simulink model "SalirClaseConObstaculos"  (R2023b)
settings: Solver=FixedStepDiscrete  StartTime=0.0  StopTime=100  FixedStep=0.01  RelTol=1e-3  EnableMultiTasking=on
model workspace (MAT data in the model file):
  baldosa = 0.48
  d = 0.2625
libraries: robotalgslib x1
settings Model: ExtModeTrigDuration=2  Creator=Usuario_UMA  LastModifiedBy=pablo
settings SolverCC: AlgebraicLoopSolver=TrustRegion
settings OptimizationCC: EnhancedBackFolding=on  PassReuseOutputArgsAs=Individual arguments  ZeroExternalMemoryAtStartup=off  ZeroInternalMemoryAtStartup=off  MaxStackSize=64  OptimizeBlockOrder=speed  DifferentSizesBufferReuse=on  EfficientTunableParamExpr=on
settings DebuggingCC: ParameterTunabilityLossMsg=error  UnconnectedInputMsg=warning  UnconnectedOutputMsg=warning  UnconnectedLineMsg=warning
settings HardwareCC: ProdBitPerInt=16  ProdBitPerPointer=16  ProdBitPerSizeT=16  ProdBitPerPtrDiffT=16  ProdLargestAtomicFloat=None  ProdWordSize=8  ProdHWDeviceType=Atmel->AVR  UseEmbeddedCoderFeatures=off  UseSimulinkCoderFeatures=off
settings ModelReferenceCC: EnableRefExpFcnMdlSchedulingChecks=on
settings SFSimCC: MATLABDynamicMemAlloc=off
settings RTWCC: Description=Embedded Coder  SystemTargetFile=ert.tlc  HardwareBoard=Arduino Mega 2560  TemplateMakefile=ert_default_tmf  Toolchain=Arduino AVR  BuildConfiguration=Faster Runs  DLArmComputeVersion=19.05
settings CodeAppCC: ForceParamTrailComments=on  IgnoreCustomStorageClasses=off  OperatorAnnotations=on  SimulinkDataObjDesc=on  SFDataObjDesc=on  InsertBlockDesc=on
settings ERTTargetCC: SupportContinuousTime=on  SupportNonInlinedSFcns=on  SupportVariableSizeSignals=on  ExtModeTransport=3  ExtModeStaticAlloc=on  ExtModeAutomaticAllocSize=off  ExtModeStaticAllocSize=2048  ExtModeMexFile=ext_xcp  ExtModeIntrfLevel=Level2 - Open

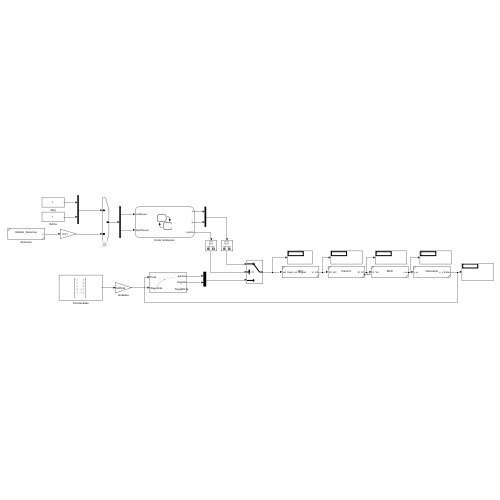
[thumbnail: Simulink's stored preview of the top-level diagram]
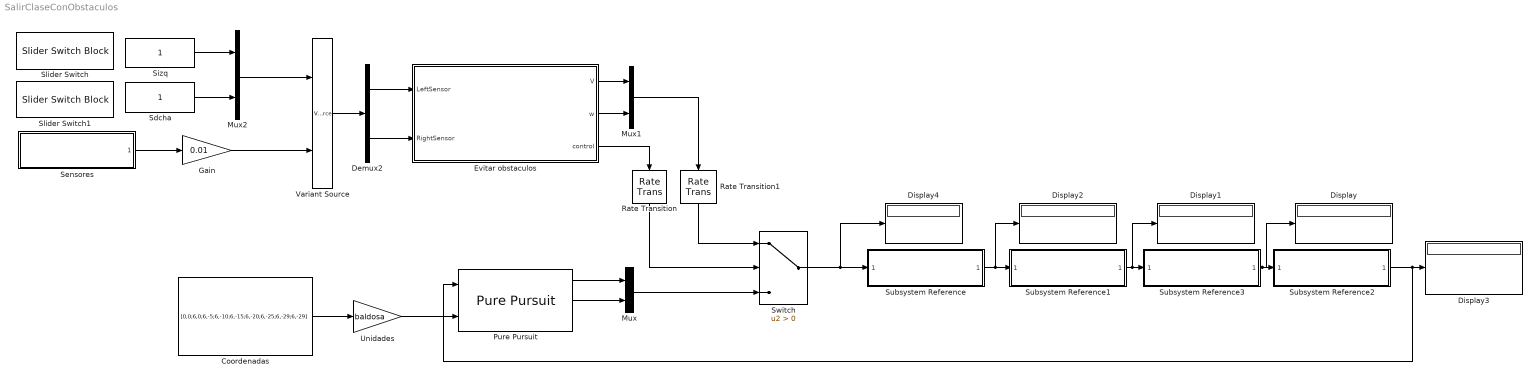
== system SalirClaseConObstaculos ==
  Coordenadas : Constant  Value=[0,0;6,0;6,-5;6,-10;6,-15;6,-20;6,-25;6,-29;6,-29]
  Demux2 : Demux  Outputs=2
  Display{,1..4} (5 alike) : Display
  Evitar obstaculos : Stateflow chart  TreatAsAtomicUnit=on
  Gain : Gain  Gain=0.01  OutDataTypeStr=double
  Mux : Mux  Inputs=2
  Mux1 : Mux  Inputs=2
  Mux2 : Mux  Inputs=2
  Pure Pursuit : robotalgslib/Pure Pursuit  DesiredLinearVelocity=0.205  MaxAngularVelocity=1.5  LookaheadDistance=0.2  TargetDirPort=on  SimulateUsing=Code generation
      settings: LibrarySourceBlock=navlib/Control Algorithms/Pure Pursuit
  Rate Transition : RateTransition
  Rate Transition1 : RateTransition
  Sdcha : Constant
  Sensores : Subsystem  ReferencedSubsystem=Modelo_Sensores
  Sizq : Constant
  Slider Switch : SliderSwitchBlock
      settings: Values={{'Libre', 'Obstaculo'}, [1 0.29]}
  Slider Switch1 : SliderSwitchBlock
      settings: Values={{'Libre', 'Obstaculo'}, [1 0.29]}
  Subsystem Reference : Subsystem  ReferencedSubsystem=MCI
  Subsystem Reference1 : Subsystem  ReferencedSubsystem=PieroCV
  Subsystem Reference2 : Subsystem  ReferencedSubsystem=Odometria
  Subsystem Reference3 : Subsystem  ReferencedSubsystem=MCD
  Switch : Switch  Criteria=u2 > Threshold  SaturateOnIntegerOverflow=off  InputSameDT=off
  Unidades : Gain  Gain=baldosa
  Variant Source : VariantSource  VariantControlMode=sim codegen switching
  wires:
  Subsystem Reference3/1 -> Display/1, Subsystem Reference2/1
  Subsystem Reference1/1 -> Display1/1, Subsystem Reference3/1
  Subsystem Reference/1 -> Display2/1, Subsystem Reference1/1
  Subsystem Reference2/1 -> Pure Pursuit/1, Display3/1
  Pure Pursuit/1 -> Mux/1
  Coordenadas/1 -> Unidades/1
  Pure Pursuit/2 -> Mux/2
  Mux/1 -> Switch/3
  Evitar obstaculos/1(V) -> Mux1/1
  Evitar obstaculos/2(w) -> Mux1/2
  Mux1/1 -> Rate Transition1/1
  Switch/1 -> Display4/1, Subsystem Reference/1
  Evitar obstaculos/3(control) -> Rate Transition/1
  Sensores/1 -> Gain/1
  Demux2/1 -> Evitar obstaculos/1(LeftSensor)
  Demux2/2 -> Evitar obstaculos/2(RightSensor)
  Rate Transition/1 -> Switch/2
  Gain/1 -> Variant Source/2
  Sdcha/1 -> Mux2/2
  Sizq/1 -> Mux2/1
  Mux2/1 -> Variant Source/1
  Variant Source/1 -> Demux2/1
  Rate Transition1/1 -> Switch/1
  Unidades/1 -> Pure Pursuit/2

== stateflow chart SalirClaseConObstaculos/Evitar obstaculos ==
  state SinObstaculos
    en:
    control = 0;
    V = 0.205;
    w = 1;
  state ObstaculoDcha
    en:
    control = 1;
    V = 0.1;
    w = 0.5;
  state ObstaculoIzq
    en:
    control = 1;
    V = 0.1;
    w = -0.5;
  state ObstaculoFrente
    en:
    control = 1;
    V = 0;
    w = 2;
  (default) -> SinObstaculos
  SinObstaculos -> ObstaculoDcha [order 2] : [RightSensor<0.3]
  SinObstaculos -> ObstaculoIzq [order 1] : [LeftSensor<0.3]
  ObstaculoIzq -> SinObstaculos [order 1] : after(3,sec)
  ObstaculoDcha -> SinObstaculos [order 1] : after(3,sec)
  ObstaculoFrente -> SinObstaculos : after(3,sec)
  ObstaculoIzq -> ObstaculoFrente [order 2] : [RightSensor<0.3]
  ObstaculoDcha -> ObstaculoFrente [order 2] : [LeftSensor<0.3]
  data: V output double size=1; w output double size=1; LeftSensor input size=1; RightSensor input size=1; control output uint8 size=1
  data V settings: description=Velocidad lineal del vehiculo
